simulink library "AMK_CAN_lib"  (R2022b)
settings: Solver=VariableStepAuto  StartTime=0.0  StopTime=10.0  RelTol=1e-3
undefined symbols (not defined in the file): canChannel
libraries: $bdroot x7, canmsglib x6, canlib x3, realtime_pacer_lib x1
settings Model: Creator=dr_pa  LastModifiedBy=dr_pa

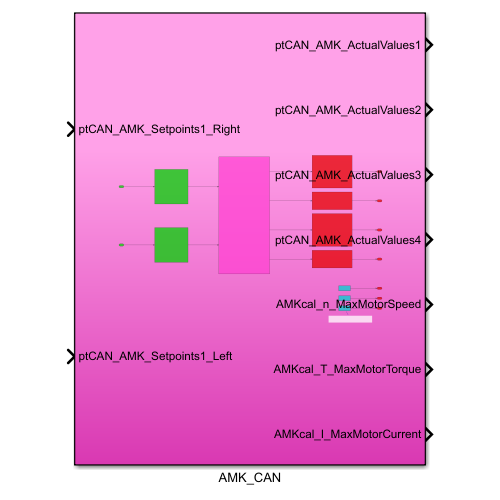
[thumbnail: Simulink's stored preview of the top-level diagram]
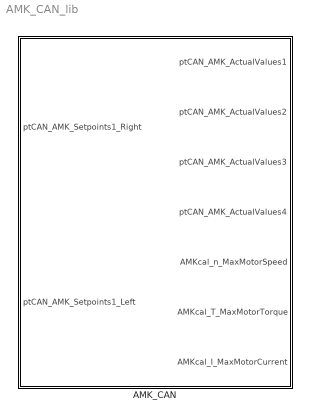
== system AMK_CAN_lib ==
  AMK_CAN : Subsystem

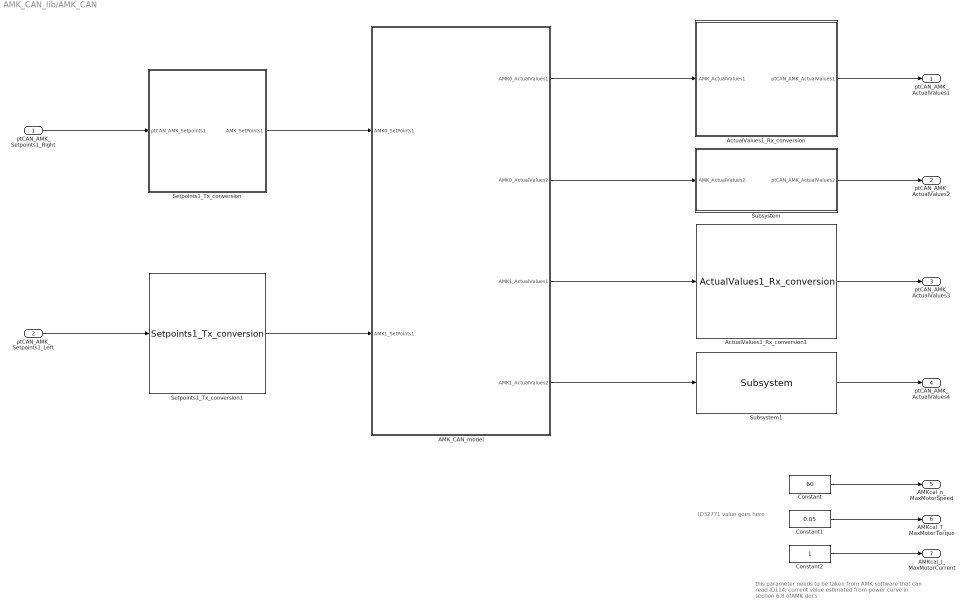
== system AMK_CAN_lib/AMK_CAN ==
  note: this parameter needs to be taken from AMK software that
      | can read ID114; current value estimated from power curve
      | in section 6.8 ofAMK docs
  note: ID32771 value goes here
  ptCAN_AMK_Setpoints1_Right : Inport
  ptCAN_AMK_Setpoints1_Left : Inport  Port=2
  AMK_CAN_model : Subsystem
  ActualValues1_Rx_conversion : Subsystem
  ActualValues1_Rx_conversion1 : $bdroot/AMK_CAN/ActualValues1_Rx_conversion  SystemSampleTime=-1  VariantActivationTime=update diagram  Latency=0  AutoFrameSizeCalculation=off
  Constant : Constant  Value=60  OutDataTypeStr=single
  Constant1 : Constant  Value=0.05  OutDataTypeStr=single
  Constant2 : Constant  OutDataTypeStr=single
  Setpoints1_Tx_conversion : Subsystem
  Setpoints1_Tx_conversion1 : $bdroot/AMK_CAN/Setpoints1_Tx_conversion  SystemSampleTime=-1  VariantActivationTime=update diagram  Latency=0  AutoFrameSizeCalculation=off
  Subsystem : Subsystem
  Subsystem1 : $bdroot/AMK_CAN/Subsystem  SystemSampleTime=-1  VariantActivationTime=update diagram  Latency=0  AutoFrameSizeCalculation=off
  ptCAN_AMK_ActualValues1 : Outport
  ptCAN_AMK_ActualValues2 : Outport  Port=2
  ptCAN_AMK_ActualValues3 : Outport  Port=3
  ptCAN_AMK_ActualValues4 : Outport  Port=4
  AMKcal_n_MaxMotorSpeed : Outport  Port=5
  AMKcal_T_MaxMotorTorque : Outport  Port=6
  AMKcal_I_MaxMotorCurrent : Outport  Port=7
  wires:
  Setpoints1_Tx_conversion1/1 -> AMK_CAN_model/2(AMK1_SetPoints1)
  ptCAN_AMK_Setpoints1_Right/1 -> Setpoints1_Tx_conversion/1(ptCAN_AMK_Setpoints1)
  AMK_CAN_model/3(AMK1_ActualValues1) -> ActualValues1_Rx_conversion1/1
  AMK_CAN_model/4(AMK1_ActualValues2) -> Subsystem1/1
  AMK_CAN_model/1(AMK0_ActualValues1) -> ActualValues1_Rx_conversion/1(AMK_ActualValues1)
  Setpoints1_Tx_conversion/1(AMK_SetPoints1) -> AMK_CAN_model/1(AMK0_SetPoints1)
  AMK_CAN_model/2(AMK0_ActualValues2) -> Subsystem/1(AMK_ActualValues2)
  ptCAN_AMK_Setpoints1_Left/1 -> Setpoints1_Tx_conversion1/1
  ActualValues1_Rx_conversion/1(ptCAN_AMK_ActualValues1) -> ptCAN_AMK_ActualValues1/1
  ActualValues1_Rx_conversion1/1 -> ptCAN_AMK_ActualValues3/1
  Subsystem/1(ptCAN_AMK_ActualValues2) -> ptCAN_AMK_ActualValues2/1
  Subsystem1/1 -> ptCAN_AMK_ActualValues4/1
  Constant/1 -> AMKcal_n_MaxMotorSpeed/1
  Constant1/1 -> AMKcal_T_MaxMotorTorque/1
  Constant2/1 -> AMKcal_I_MaxMotorCurrent/1

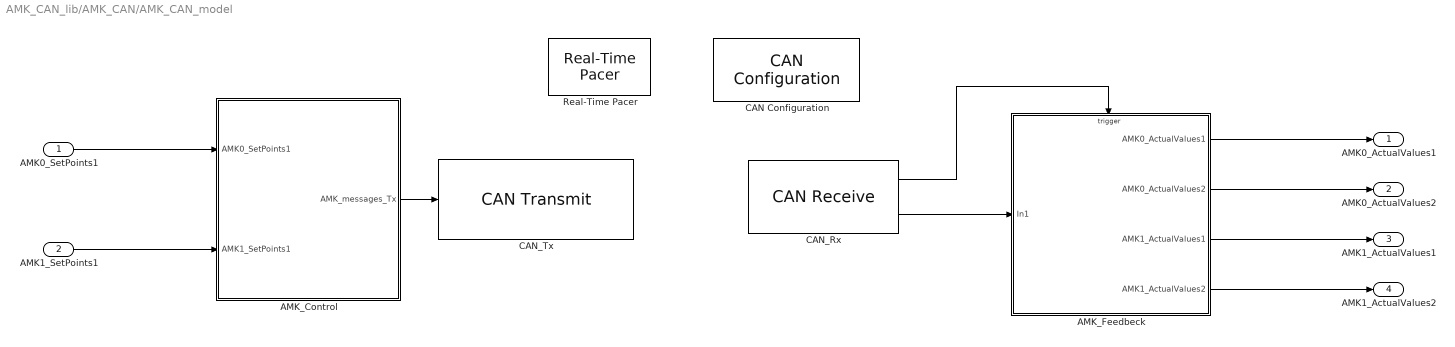
== system AMK_CAN_lib/AMK_CAN/AMK_CAN_model ==
  AMK0_SetPoints1 : Inport
  AMK1_SetPoints1 : Inport  Port=2
  AMK_Control : Subsystem
  AMK_Feedbeck : Subsystem  TreatAsAtomicUnit=on
  CAN Configuration : canlib/CAN Configuration  BlockHandle=4897.0001  Device=MathWorks Virtual 1 (Channel 1)  DeviceMenu=MathWorks Virtual 1 (Channel 1)  ObjConstructor=canChannel('MathWorks', 'Virtual 1', 1)  BusSpeed=500000  EnableBitParameters=off  AckMode=Normal
  CAN_Rx : canlib/CAN Receive  BlockHandle=4898.0001  Device=MathWorks Virtual 1 (Channel 1)  DeviceMenu=MathWorks Virtual 1 (Channel 1)  ObjConstructor=canChannel('MathWorks', 'Virtual 1', 1)  EnableStandardIDsFilter=off  StdIDsCombo=Allow all  StandardIDs=0  EnableExtendedIDsFilter=off  ExtIDsCombo=Allow all  ExtendedIDs=0  SampleTime=0.005  MsgsPerTimestep=all  InternalFilterUpdateStatus=on  BusOutput=off
  CAN_Tx : canlib/CAN Transmit  BlockHandle=4901.0001  Device=MathWorks Virtual 1 (Channel 1)  DeviceMenu=MathWorks Virtual 1 (Channel 1)  ObjConstructor=canChannel('MathWorks', 'Virtual 1', 1)  EnableEventTransmit=off  EnablePeriodicTransmit=on  MessagePeriod=0.01
  Real-Time Pacer : realtime_pacer_lib/Real-Time Pacer  simTimePerRealTime=1
  AMK0_ActualValues1 : Outport
  AMK0_ActualValues2 : Outport  Port=2
  AMK1_ActualValues1 : Outport  Port=3
  AMK1_ActualValues2 : Outport  Port=4
  wires:
  CAN_Rx/2 -> AMK_Feedbeck/1(In1)
  AMK_Feedbeck/1(AMK0_ActualValues1) -> AMK0_ActualValues1/1
  AMK0_SetPoints1/1 -> AMK_Control/1(AMK0_SetPoints1)
  AMK_Control/1(AMK_messages_Tx) -> CAN_Tx/1
  CAN_Rx/1 -> AMK_Feedbeck/Trigger
  AMK_Feedbeck/2(AMK0_ActualValues2) -> AMK0_ActualValues2/1
  AMK_Feedbeck/4(AMK1_ActualValues2) -> AMK1_ActualValues2/1
  AMK_Feedbeck/3(AMK1_ActualValues1) -> AMK1_ActualValues1/1
  AMK1_SetPoints1/1 -> AMK_Control/2(AMK1_SetPoints1)

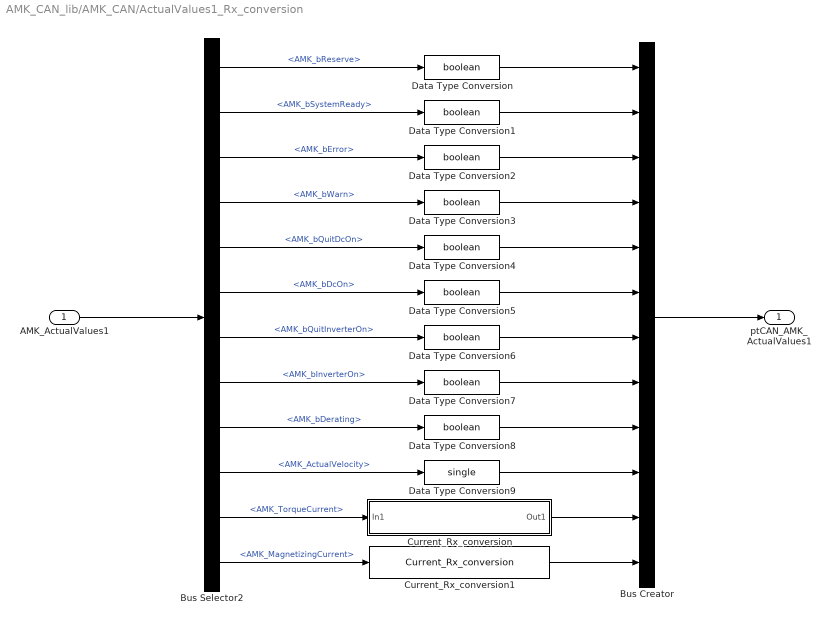
== system AMK_CAN_lib/AMK_CAN/ActualValues1_Rx_conversion ==
  AMK_ActualValues1 : Inport
  Bus Creator : BusCreator  Inputs=12
  Bus Selector2 : BusSelector  OutputSignals=AMK_bReserve,AMK_bSystemReady,AMK_bError,AMK_bWarn,AMK_bQuitDcOn,AMK_bDcOn,AMK_bQuitInverterOn,AMK_bInverterOn,AMK_bDerating,AMK_ActualVelocity,AMK_TorqueCurrent,AMK_MagnetizingCurrent
  Current_Rx_conversion : Subsystem
  Current_Rx_conversion1 : $bdroot/AMK_CAN/ActualValues1_Rx_conversion/Current_Rx_conversion  SystemSampleTime=-1  VariantActivationTime=update diagram  Latency=0  AutoFrameSizeCalculation=off
  Data Type Conversion{,1..8} (9 alike) : DataTypeConversion  OutDataTypeStr=boolean  SaturateOnIntegerOverflow=off  RndMeth=Floor
  Data Type Conversion9 : DataTypeConversion  OutDataTypeStr=single  SaturateOnIntegerOverflow=off  RndMeth=Floor
  ptCAN_AMK_ActualValues1 : Outport
  wires:
  Bus Selector2/5 -> Data Type Conversion4/1  "<AMK_bQuitDcOn>"
  Bus Selector2/9 -> Data Type Conversion8/1  "<AMK_bDerating>"
  Bus Selector2/6 -> Data Type Conversion5/1  "<AMK_bDcOn>"
  Bus Selector2/4 -> Data Type Conversion3/1  "<AMK_bWarn>"
  Bus Selector2/1 -> Data Type Conversion/1  "<AMK_bReserve>"
  Bus Selector2/11 -> Current_Rx_conversion/1(In1)  "<AMK_TorqueCurrent>"
  Bus Selector2/12 -> Current_Rx_conversion1/1  "<AMK_MagnetizingCurrent>"
  Bus Selector2/8 -> Data Type Conversion7/1  "<AMK_bInverterOn>"
  Bus Selector2/7 -> Data Type Conversion6/1  "<AMK_bQuitInverterOn>"
  Bus Selector2/2 -> Data Type Conversion1/1  "<AMK_bSystemReady>"
  Bus Selector2/3 -> Data Type Conversion2/1  "<AMK_bError>"
  Bus Selector2/10 -> Data Type Conversion9/1  "<AMK_ActualVelocity>"
  AMK_ActualValues1/1 -> Bus Selector2/1
  Bus Creator/1 -> ptCAN_AMK_ActualValues1/1
  Data Type Conversion/1 -> Bus Creator/1
  Data Type Conversion1/1 -> Bus Creator/2
  Data Type Conversion2/1 -> Bus Creator/3
  Data Type Conversion3/1 -> Bus Creator/4
  Data Type Conversion4/1 -> Bus Creator/5
  Data Type Conversion5/1 -> Bus Creator/6
  Data Type Conversion6/1 -> Bus Creator/7
  Data Type Conversion7/1 -> Bus Creator/8
  Data Type Conversion8/1 -> Bus Creator/9
  Data Type Conversion9/1 -> Bus Creator/10
  Current_Rx_conversion/1(Out1) -> Bus Creator/11
  Current_Rx_conversion1/1 -> Bus Creator/12

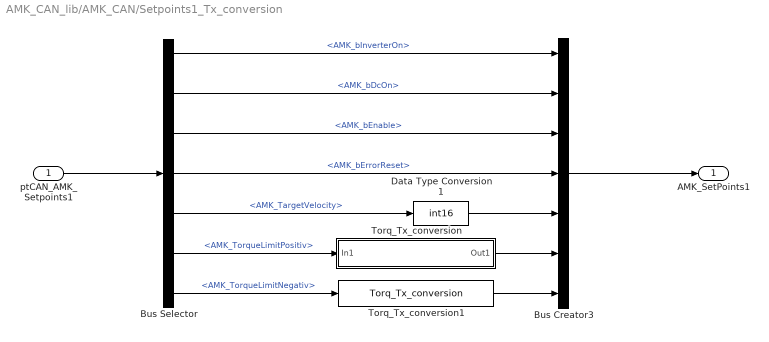
== system AMK_CAN_lib/AMK_CAN/Setpoints1_Tx_conversion ==
  ptCAN_AMK_Setpoints1 : Inport
  Bus Creator3 : BusCreator  Inputs=7
  Bus Selector : BusSelector  OutputSignals=AMK_bInverterOn,AMK_bDcOn,AMK_bEnable,AMK_bErrorReset,AMK_TargetVelocity,AMK_TorqueLimitPositiv,AMK_TorqueLimitNegativ
  Data Type Conversion1 : DataTypeConversion  OutDataTypeStr=int16  SaturateOnIntegerOverflow=off  RndMeth=Floor
  Torq_Tx_conversion : Subsystem
  Torq_Tx_conversion1 : $bdroot/AMK_CAN/Setpoints1_Tx_conversion/Torq_Tx_conversion  SystemSampleTime=-1  VariantActivationTime=update diagram  Latency=0  AutoFrameSizeCalculation=off
  AMK_SetPoints1 : Outport
  wires:
  Bus Selector/4 -> Bus Creator3/4  "<AMK_bErrorReset>"
  Data Type Conversion1/1 -> Bus Creator3/5
  Bus Selector/3 -> Bus Creator3/3  "<AMK_bEnable>"
  Torq_Tx_conversion1/1 -> Bus Creator3/7
  Bus Selector/6 -> Torq_Tx_conversion/1(In1)  "<AMK_TorqueLimitPositiv>"
  Bus Selector/2 -> Bus Creator3/2  "<AMK_bDcOn>"
  Bus Selector/5 -> Data Type Conversion1/1  "<AMK_TargetVelocity>"
  Bus Selector/1 -> Bus Creator3/1  "<AMK_bInverterOn>"
  Bus Creator3/1 -> AMK_SetPoints1/1
  Bus Selector/7 -> Torq_Tx_conversion1/1  "<AMK_TorqueLimitNegativ>"
  Torq_Tx_conversion/1(Out1) -> Bus Creator3/6
  ptCAN_AMK_Setpoints1/1 -> Bus Selector/1

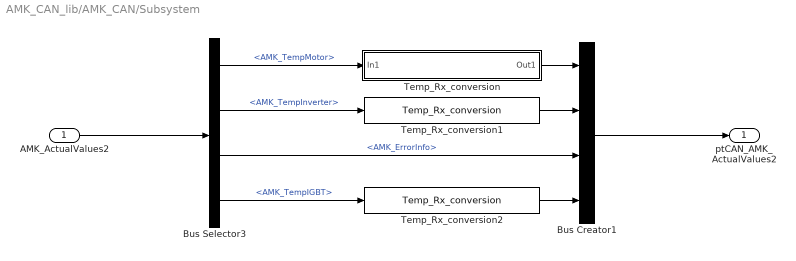
== system AMK_CAN_lib/AMK_CAN/Subsystem ==
  AMK_ActualValues2 : Inport
  Bus Creator1 : BusCreator  Inputs=4
  Bus Selector3 : BusSelector  OutputSignals=AMK_TempMotor,AMK_TempInverter,AMK_ErrorInfo,AMK_TempIGBT
  Temp_Rx_conversion : Subsystem
  Temp_Rx_conversion1 : $bdroot/AMK_CAN/Subsystem/Temp_Rx_conversion  SystemSampleTime=-1  VariantActivationTime=update diagram  Latency=0  AutoFrameSizeCalculation=off
  Temp_Rx_conversion2 : $bdroot/AMK_CAN/Subsystem/Temp_Rx_conversion  SystemSampleTime=-1  VariantActivationTime=update diagram  Latency=0  AutoFrameSizeCalculation=off
  ptCAN_AMK_ActualValues2 : Outport
  wires:
  Bus Selector3/4 -> Temp_Rx_conversion2/1  "<AMK_TempIGBT>"
  Bus Selector3/1 -> Temp_Rx_conversion/1(In1)  "<AMK_TempMotor>"
  Bus Selector3/3 -> Bus Creator1/3  "<AMK_ErrorInfo>"
  Bus Creator1/1 -> ptCAN_AMK_ActualValues2/1
  AMK_ActualValues2/1 -> Bus Selector3/1
  Bus Selector3/2 -> Temp_Rx_conversion1/1  "<AMK_TempInverter>"
  Temp_Rx_conversion/1(Out1) -> Bus Creator1/1
  Temp_Rx_conversion1/1 -> Bus Creator1/2
  Temp_Rx_conversion2/1 -> Bus Creator1/4

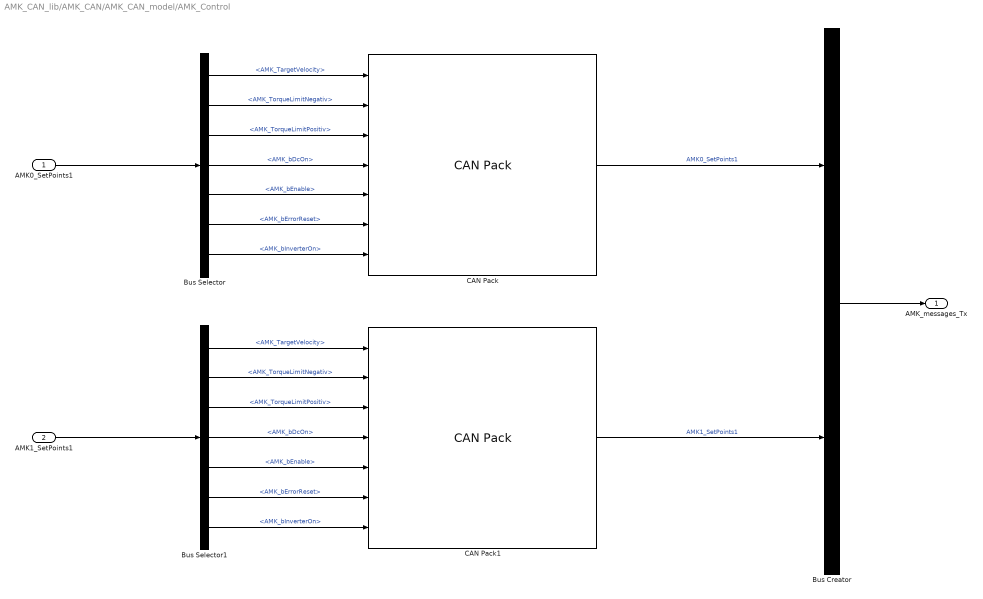
== system AMK_CAN_lib/AMK_CAN/AMK_CAN_model/AMK_Control ==
  AMK0_SetPoints1 : Inport
  AMK1_SetPoints1 : Inport  Port=2
  Bus Creator : BusCreator  Inputs=2
  Bus Selector : BusSelector  OutputSignals=ptCAN_AMK_Setpoints1_Right.AMK_TargetVelocity,ptCAN_AMK_Setpoints1_Right.AMK_TorqueLimitNegativ,ptCAN_AMK_Setpoints1_Right.AMK_TorqueLimitPositiv,ptCAN_AMK_Setpoints1_Right.AMK_bDcOn,ptCAN_AMK_Setpoints1_Right.AMK_bEnable,ptCAN_AMK_Setpoints1_Right.AMK_bErrorReset,ptCAN_AMK_Setpoints1_Right.AMK_bInverterOn
  Bus Selector1 : BusSelector  OutputSignals=ptCAN_AMK_Setpoints1_Right.AMK_TargetVelocity,ptCAN_AMK_Setpoints1_Right.AMK_TorqueLimitNegativ,ptCAN_AMK_Setpoints1_Right.AMK_TorqueLimitPositiv,ptCAN_AMK_Setpoints1_Right.AMK_bDcOn,ptCAN_AMK_Setpoints1_Right.AMK_bEnable,ptCAN_AMK_Setpoints1_Right.AMK_bErrorReset,ptCAN_AMK_Setpoints1_Right.AMK_bInverterOn
  CAN Pack : canmsglib/CAN Pack  CANdbFile=C:\Users\dr_pa\git\school\vehicle_control_system\src\Plant\Bench\CAN_Databases-master\CAN_AMKInverter.dbc  MsgList=AMK0_SetPoints1  MsgName=AMK0_SetPoints1  MsgIDType=Standard (11-bit identifier)  MsgIdentifier=389  MsgLength=8  Remote=off  ApplyMinMax=off  BusOutput=off  SignalInfo={'AMK_TargetVelocity','16','16','LE','signed','Standard','0','1','0','-Inf','Inf';'AMK_TorqueLimitNegativ','48','16','LE','signed','Standard','0','1','0','-Inf','Inf';'AMK_TorqueLimitPositiv','32','16','LE','signed','Standard','0','1','0','-Inf','Inf';'AMK_bDcOn','9','1','LE','unsigned','Standard','0','1','0','-Inf','Inf';'AMK_bEnable','10','1','LE','unsigned','Standard','0','1','0','-Inf','Inf';'AMK_bErrorReset','11','1','LE','unsigned','Standard','0','1','0','-Inf','Inf';'AMK_bInverterOn','8','1','LE','unsigned','Standard','0','1','0','-Inf','Inf'}
      settings: LibrarySourceBlock=canlib/CAN Pack  DataFormat=CANdb specified signals
  CAN Pack1 : canmsglib/CAN Pack  CANdbFile=C:\Users\dr_pa\git\school\vehicle_control_system\src\Plant\Bench\CAN_Databases-master\CAN_AMKInverter.dbc  MsgList=AMK1_SetPoints1  MsgName=AMK1_SetPoints1  MsgIDType=Standard (11-bit identifier)  MsgIdentifier=390  MsgLength=8  Remote=off  ApplyMinMax=off  BusOutput=off  SignalInfo={'AMK_TargetVelocity','16','16','LE','signed','Standard','0','1','0','-Inf','Inf';'AMK_TorqueLimitNegativ','48','16','LE','signed','Standard','0','1','0','-Inf','Inf';'AMK_TorqueLimitPositiv','32','16','LE','signed','Standard','0','1','0','-Inf','Inf';'AMK_bDcOn','9','1','LE','unsigned','Standard','0','1','0','-Inf','Inf';'AMK_bEnable','10','1','LE','unsigned','Standard','0','1','0','-Inf','Inf';'AMK_bErrorReset','11','1','LE','unsigned','Standard','0','1','0','-Inf','Inf';'AMK_bInverterOn','8','1','LE','unsigned','Standard','0','1','0','-Inf','Inf'}
      settings: LibrarySourceBlock=canlib/CAN Pack  DataFormat=CANdb specified signals
  AMK_messages_Tx : Outport
  wires:
  AMK0_SetPoints1/1 -> Bus Selector/1
  CAN Pack/1 -> Bus Creator/1  "AMK0_SetPoints1"
  CAN Pack1/1 -> Bus Creator/2  "AMK1_SetPoints1"
  Bus Creator/1 -> AMK_messages_Tx/1
  Bus Selector/7 -> CAN Pack/7  "<AMK_bInverterOn>"
  Bus Selector/4 -> CAN Pack/4  "<AMK_bDcOn>"
  Bus Selector/5 -> CAN Pack/5  "<AMK_bEnable>"
  Bus Selector/6 -> CAN Pack/6  "<AMK_bErrorReset>"
  Bus Selector/1 -> CAN Pack/1  "<AMK_TargetVelocity>"
  Bus Selector1/1 -> CAN Pack1/1  "<AMK_TargetVelocity>"
  Bus Selector1/6 -> CAN Pack1/6  "<AMK_bErrorReset>"
  Bus Selector1/5 -> CAN Pack1/5  "<AMK_bEnable>"
  Bus Selector1/4 -> CAN Pack1/4  "<AMK_bDcOn>"
  Bus Selector1/7 -> CAN Pack1/7  "<AMK_bInverterOn>"
  AMK1_SetPoints1/1 -> Bus Selector1/1
  Bus Selector/2 -> CAN Pack/2  "<AMK_TorqueLimitNegativ>"
  Bus Selector/3 -> CAN Pack/3  "<AMK_TorqueLimitPositiv>"
  Bus Selector1/2 -> CAN Pack1/2  "<AMK_TorqueLimitNegativ>"
  Bus Selector1/3 -> CAN Pack1/3  "<AMK_TorqueLimitPositiv>"

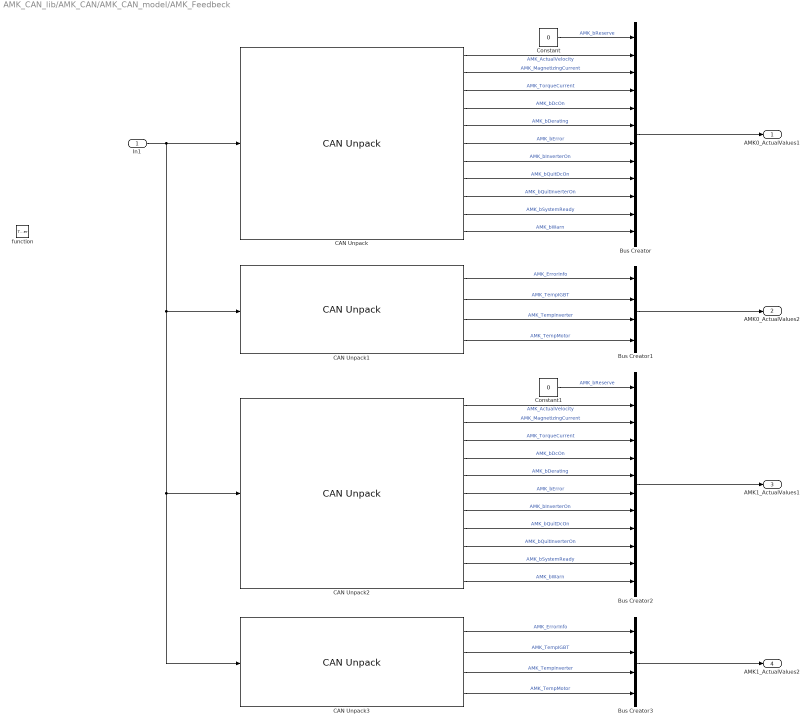
== system AMK_CAN_lib/AMK_CAN/AMK_CAN_model/AMK_Feedbeck ==
  In1 : Inport
  function : TriggerPort  TriggerType=function-call  VariantControl=(inherit)
  Bus Creator : BusCreator  Inputs=12
  Bus Creator1 : BusCreator  Inputs=4
  Bus Creator2 : BusCreator  Inputs=12
  Bus Creator3 : BusCreator  Inputs=4
  CAN Unpack : canmsglib/CAN Unpack  CANdbFile=C:\Users\dr_pa\git\school\vehicle_control_system\src\Plant\Bench\CAN_Databases-master\CAN_AMKInverter.dbc  MsgList=AMK0_ActualValues1  MsgName=AMK0_ActualValues1  MsgIDType=Standard (11-bit identifier)  MsgIdentifier=644  MsgLength=8  SignalInfo={'AMK_ActualVelocity','16','16','LE','signed','Standard','0','1','0','-Inf','Inf';'AMK_MagnetizingCurrent','48','16','LE','signed','Standard','0','1','0','-Inf','Inf';'AMK_TorqueCurrent','32','16','LE','signed','Standard','0','1','0','-Inf','Inf';'AMK_bDcOn','12','1','LE','unsigned','Standard','0','1','0','-Inf','Inf';'AMK_bDerating','15','1','LE','unsigned','Standard','0','1','0','-Inf','Inf';'AMK_bError','9','1','LE','unsigned','Standard','0','1','0','-Inf','Inf';'AMK_bInverterOn','14','1','LE','unsigned','Standard','0','1','0','-Inf','Inf';'AMK_bQuitDcOn','11','1','LE','unsigned','Standard','0','1','0','-Inf','Inf';'AMK_bQuitInverterOn','13','1','LE','unsigned','Standard','0','1','0','-Inf','Inf';'AMK_bSystemReady','8','1','LE','unsigned','Standard','0','1','0','-Inf','Inf';'AMK_bWarn','10','1','LE','unsigned','Standard','0','1','0','-Inf','Inf'}  IDPort=off  TimestampPort=off  ErrorPort=off  RemotePort=off  LengthPort=off  StatusPort=off  ApplyMinMax=off
      settings: LibrarySourceBlock=canlib/CAN Unpack  DataFormat=CANdb specified signals
  CAN Unpack1 : canmsglib/CAN Unpack  CANdbFile=C:\Users\dr_pa\git\school\vehicle_control_system\src\Plant\Bench\CAN_Databases-master\CAN_AMKInverter.dbc  MsgList=AMK0_ActualValues2  MsgName=AMK0_ActualValues2  MsgIDType=Standard (11-bit identifier)  MsgIdentifier=646  MsgLength=8  SignalInfo={'AMK_ErrorInfo','32','16','LE','unsigned','Standard','0','1','0','0','65535';'AMK_TempIGBT','48','16','LE','signed','Standard','0','0.1','0','-3276.8','3276.7';'AMK_TempInverter','16','16','LE','signed','Standard','0','0.1','0','-3276.8','3276.7';'AMK_TempMotor','0','16','LE','signed','Standard','0','0.1','0','-3276.8','3276.7'}  IDPort=off  TimestampPort=off  ErrorPort=off  RemotePort=off  LengthPort=off  StatusPort=off  ApplyMinMax=off
      settings: LibrarySourceBlock=canlib/CAN Unpack  DataFormat=CANdb specified signals
  CAN Unpack2 : canmsglib/CAN Unpack  CANdbFile=C:\Users\dr_pa\git\school\vehicle_control_system\src\Plant\Bench\CAN_Databases-master\CAN_AMKInverter.dbc  MsgList=AMK1_ActualValues1  MsgName=AMK1_ActualValues1  MsgIDType=Standard (11-bit identifier)  MsgIdentifier=645  MsgLength=8  SignalInfo={'AMK_ActualVelocity','16','16','LE','signed','Standard','0','1','0','-Inf','Inf';'AMK_MagnetizingCurrent','48','16','LE','signed','Standard','0','1','0','-Inf','Inf';'AMK_TorqueCurrent','32','16','LE','signed','Standard','0','1','0','-Inf','Inf';'AMK_bDcOn','12','1','LE','unsigned','Standard','0','1','0','-Inf','Inf';'AMK_bDerating','15','1','LE','unsigned','Standard','0','1','0','-Inf','Inf';'AMK_bError','9','1','LE','unsigned','Standard','0','1','0','-Inf','Inf';'AMK_bInverterOn','14','1','LE','unsigned','Standard','0','1','0','-Inf','Inf';'AMK_bQuitDcOn','11','1','LE','unsigned','Standard','0','1','0','-Inf','Inf';'AMK_bQuitInverterOn','13','1','LE','unsigned','Standard','0','1','0','-Inf','Inf';'AMK_bSystemReady','8','1','LE','unsigned','Standard','0','1','0','-Inf','Inf';'AMK_bWarn','10','1','LE','unsigned','Standard','0','1','0','-Inf','Inf'}  IDPort=off  TimestampPort=off  ErrorPort=off  RemotePort=off  LengthPort=off  StatusPort=off  ApplyMinMax=off
      settings: LibrarySourceBlock=canlib/CAN Unpack  DataFormat=CANdb specified signals
  CAN Unpack3 : canmsglib/CAN Unpack  CANdbFile=C:\Users\dr_pa\git\school\vehicle_control_system\src\Plant\Bench\CAN_Databases-master\CAN_AMKInverter.dbc  MsgList=AMK1_ActualValues2  MsgName=AMK1_ActualValues2  MsgIDType=Standard (11-bit identifier)  MsgIdentifier=647  MsgLength=8  SignalInfo={'AMK_ErrorInfo','32','16','LE','unsigned','Standard','0','1','0','0','65535';'AMK_TempIGBT','48','16','LE','signed','Standard','0','0.1','0','-3276.8','3276.7';'AMK_TempInverter','16','16','LE','signed','Standard','0','0.1','0','-3276.8','3276.7';'AMK_TempMotor','0','16','LE','signed','Standard','0','0.1','0','-3276.8','3276.7'}  IDPort=off  TimestampPort=off  ErrorPort=off  RemotePort=off  LengthPort=off  StatusPort=off  ApplyMinMax=off
      settings: LibrarySourceBlock=canlib/CAN Unpack  DataFormat=CANdb specified signals
  Constant : Constant  Value=0  OutDataTypeStr=boolean
  Constant1 : Constant  Value=0  OutDataTypeStr=boolean
  AMK0_ActualValues1 : Outport
  AMK0_ActualValues2 : Outport  Port=2
  AMK1_ActualValues1 : Outport  Port=3
  AMK1_ActualValues2 : Outport  Port=4
  wires:
  In1/1 -> CAN Unpack3/1, CAN Unpack2/1, CAN Unpack1/1, CAN Unpack/1
  CAN Unpack/1 -> Bus Creator/2  "AMK_ActualVelocity"
  CAN Unpack/2 -> Bus Creator/3  "AMK_MagnetizingCurrent"
  CAN Unpack/3 -> Bus Creator/4  "AMK_TorqueCurrent"
  CAN Unpack/4 -> Bus Creator/5  "AMK_bDcOn"
  CAN Unpack/5 -> Bus Creator/6  "AMK_bDerating"
  CAN Unpack/6 -> Bus Creator/7  "AMK_bError"
  CAN Unpack/7 -> Bus Creator/8  "AMK_bInverterOn"
  CAN Unpack/8 -> Bus Creator/9  "AMK_bQuitDcOn"
  CAN Unpack/9 -> Bus Creator/10  "AMK_bQuitInverterOn"
  CAN Unpack/10 -> Bus Creator/11  "AMK_bSystemReady"
  CAN Unpack/11 -> Bus Creator/12  "AMK_bWarn"
  Bus Creator/1 -> AMK0_ActualValues1/1
  CAN Unpack2/1 -> Bus Creator2/2  "AMK_ActualVelocity"
  CAN Unpack2/10 -> Bus Creator2/11  "AMK_bSystemReady"
  CAN Unpack2/6 -> Bus Creator2/7  "AMK_bError"
  CAN Unpack2/9 -> Bus Creator2/10  "AMK_bQuitInverterOn"
  CAN Unpack2/2 -> Bus Creator2/3  "AMK_MagnetizingCurrent"
  CAN Unpack2/3 -> Bus Creator2/4  "AMK_TorqueCurrent"
  Bus Creator2/1 -> AMK1_ActualValues1/1
  CAN Unpack2/8 -> Bus Creator2/9  "AMK_bQuitDcOn"
  CAN Unpack2/4 -> Bus Creator2/5  "AMK_bDcOn"
  CAN Unpack2/5 -> Bus Creator2/6  "AMK_bDerating"
  CAN Unpack2/11 -> Bus Creator2/12  "AMK_bWarn"
  CAN Unpack2/7 -> Bus Creator2/8  "AMK_bInverterOn"
  CAN Unpack1/1 -> Bus Creator1/1  "AMK_ErrorInfo"
  CAN Unpack1/2 -> Bus Creator1/2  "AMK_TempIGBT"
  CAN Unpack1/3 -> Bus Creator1/3  "AMK_TempInverter"
  CAN Unpack1/4 -> Bus Creator1/4  "AMK_TempMotor"
  CAN Unpack3/1 -> Bus Creator3/1  "AMK_ErrorInfo"
  CAN Unpack3/4 -> Bus Creator3/4  "AMK_TempMotor"
  Bus Creator3/1 -> AMK1_ActualValues2/1
  CAN Unpack3/3 -> Bus Creator3/3  "AMK_TempInverter"
  CAN Unpack3/2 -> Bus Creator3/2  "AMK_TempIGBT"
  Constant/1 -> Bus Creator/1  "AMK_bReserve"
  Constant1/1 -> Bus Creator2/1  "AMK_bReserve"
  Bus Creator1/1 -> AMK0_ActualValues2/1

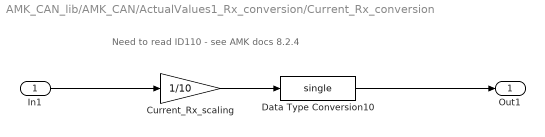
== system AMK_CAN_lib/AMK_CAN/ActualValues1_Rx_conversion/Current_Rx_conversion ==
  note: Need to read ID110 - see AMK docs 8.2.4
  In1 : Inport
  Current_Rx_scaling : Gain  Gain=1/10
  Data Type Conversion10 : DataTypeConversion  OutDataTypeStr=single  SaturateOnIntegerOverflow=off  RndMeth=Floor
  Out1 : Outport
  wires:
  Current_Rx_scaling/1 -> Data Type Conversion10/1
  In1/1 -> Current_Rx_scaling/1
  Data Type Conversion10/1 -> Out1/1

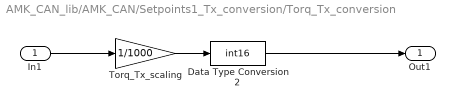
== system AMK_CAN_lib/AMK_CAN/Setpoints1_Tx_conversion/Torq_Tx_conversion ==
  In1 : Inport
  Data Type Conversion2 : DataTypeConversion  OutDataTypeStr=int16  SaturateOnIntegerOverflow=off  RndMeth=Floor
  Torq_Tx_scaling : Gain  Gain=1/1000
  Out1 : Outport
  wires:
  In1/1 -> Torq_Tx_scaling/1
  Data Type Conversion2/1 -> Out1/1
  Torq_Tx_scaling/1 -> Data Type Conversion2/1

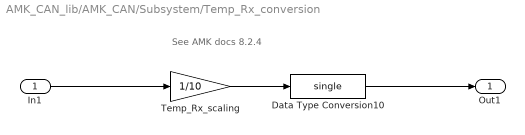
== system AMK_CAN_lib/AMK_CAN/Subsystem/Temp_Rx_conversion ==
  note: See AMK docs 8.2.4
  In1 : Inport
  Data Type Conversion10 : DataTypeConversion  OutDataTypeStr=single  SaturateOnIntegerOverflow=off  RndMeth=Floor
  Temp_Rx_scaling : Gain  Gain=1/10
  Out1 : Outport
  wires:
  In1/1 -> Temp_Rx_scaling/1
  Temp_Rx_scaling/1 -> Data Type Conversion10/1
  Data Type Conversion10/1 -> Out1/1
